simulink model "CTRL_LO_ST1_DFLATLGT_test"  (R2023b)
settings: Solver=VariableStepAuto  StartTime=0.0  StopTime=10.0  RelTol=1e-3
libraries: CTRL_LO_ST1_DFLATLGT x1
settings Model: Creator=blatak  LastModifiedBy=blatak

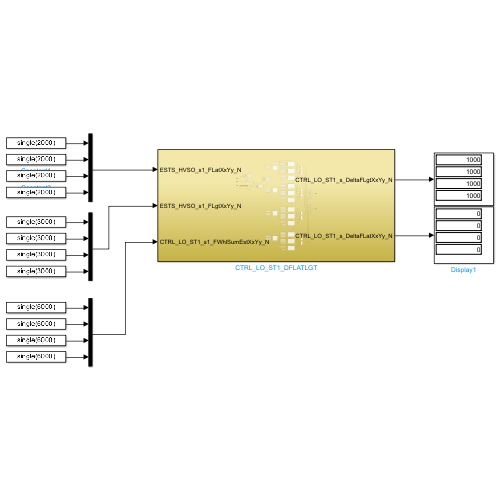
[thumbnail: Simulink's stored preview of the top-level diagram]
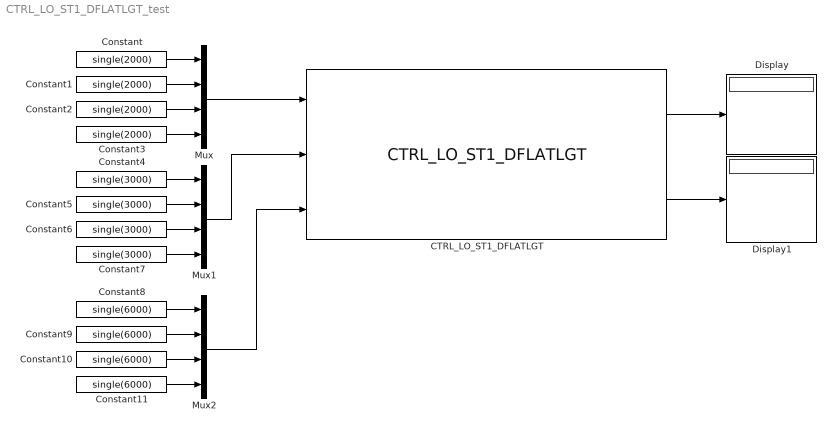
== system CTRL_LO_ST1_DFLATLGT_test ==
  CTRL_LO_ST1_DFLATLGT : CTRL_LO_ST1_DFLATLGT/CTRL_LO_ST1_DFLATLGT  SystemSampleTime=-1  VariantActivationTime=update diagram  AllowFlexibleInterface=on  Latency=0  AutoFrameSizeCalculation=off
  Constant{,1..3} (4 alike) : Constant  Value=single(2000)
  Constant{8..11} (4 alike) : Constant  Value=single(6000)
  Constant{4..7} (4 alike) : Constant  Value=single(3000)
  Display : Display
  Display1 : Display
  Mux : Mux
  Mux1 : Mux
  Mux2 : Mux
  wires:
  Constant/1 -> Mux/1
  Constant1/1 -> Mux/2
  Constant2/1 -> Mux/3
  Constant3/1 -> Mux/4
  Constant4/1 -> Mux1/1
  Constant5/1 -> Mux1/2
  Constant6/1 -> Mux1/3
  Constant7/1 -> Mux1/4
  Constant8/1 -> Mux2/1
  Constant9/1 -> Mux2/2
  Constant10/1 -> Mux2/3
  Constant11/1 -> Mux2/4
  Mux2/1 -> CTRL_LO_ST1_DFLATLGT/3
  Mux1/1 -> CTRL_LO_ST1_DFLATLGT/2
  Mux/1 -> CTRL_LO_ST1_DFLATLGT/1
  CTRL_LO_ST1_DFLATLGT/1 -> Display/1
  CTRL_LO_ST1_DFLATLGT/2 -> Display1/1
